simulink model "lidar_webcam_Bayes"  (Simulink 7.3)
settings: Solver=FixedStepDiscrete  StartTime=0.0  StopTime=inf  MaxStep=0.2  RelTol=1e-3
libraries: dspmtrx3 x2, simulink x1, vipstatistics x1, dspstat3 x1
(part 1 of 2)
settings Model: Creator=gclayton  LastModifiedBy=wildcat
settings DebuggingCC: InheritedTsInSrcMsg=none
settings RTWCC: SystemTargetFile=rlnx.tlc  GenCodeOnly=on  TemplateMakefile=rlnx_ubuntu.tmf  Description=Linux Real-Time Target  ProcessScript=rlnx_make_rtw_hook
settings RTWCC: CustomInclude=|
  | /usr/local/include/opencv/
  | /usr/local/include/
settings CodeAppCC: GenerateComments=off  SimulinkBlockComments=off
settings STFCustomTargetCC: ModelReferenceCompliant=off  MatFileLogging=on  SystemTargetFile=rlnx.tlc
settings GRTTargetCC: ModelReferenceCompliant=off  ParMdlRefBuildCompliant=off  CompOptLevelCompliant=off
settings CustomProperty: DataType=string  Value=-lm -ldl /usr/local/lib/libopencv_highgui.so.2.4 /usr/local/lib/libopencv_core.so.2.4 /usr/local/lib/libopencv_imgproc.so.2.4 -lc_urg -lc_urg_connection -lc_urg_system -lphidget21
settings EnumStrPairs: String=PC

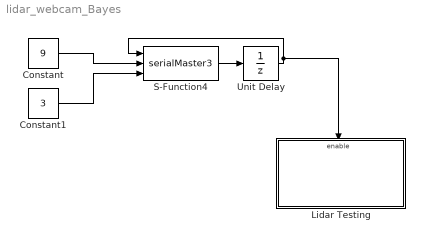
== system lidar_webcam_Bayes ==
  Constant : Constant  Value=9  OutDataTypeMode=int32  OutDataType=fixdt(1, 16)  OutScaling=2^0  OutDataTypeStr=int32
  Constant1 : Constant  Value=3  OutDataTypeMode=int32  OutDataType=fixdt(1, 16)  OutScaling=2^0  OutDataTypeStr=int32
  Lidar Testing : Subsystem  TreatAsAtomicUnit=on
  S-Function4 : S-Function  FunctionName=serialMaster3  EnableBusSupport=off
  Unit Delay : UnitDelay  SampleTime=-1
  wires:
  Constant1/1 -> S-Function4/3
  Constant/1 -> S-Function4/2
  S-Function4/1 -> Unit Delay/1
  Unit Delay/1 -> S-Function4/1, Lidar Testing/Enable

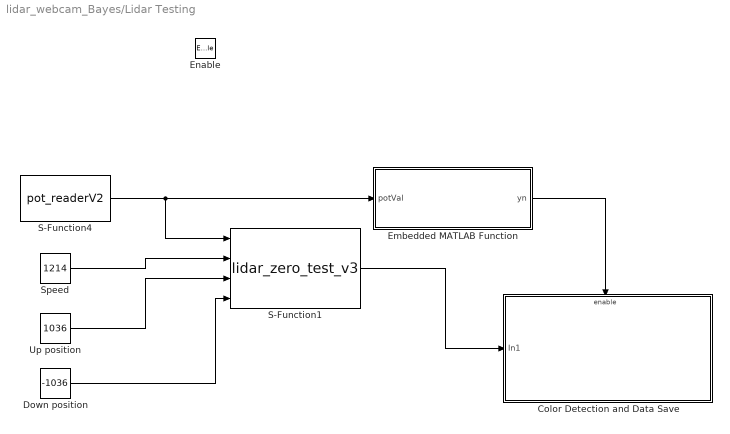
== system lidar_webcam_Bayes/Lidar Testing ==
  Enable : EnablePort
  Color Detection and Data Save : Subsystem  TreatAsAtomicUnit=on
  Down position : Constant  Value=-1036  OutDataType=fixdt(1, 16)  OutScaling=2^0
  Embedded MATLAB Function : Stateflow chart
  S-Function1 : S-Function  FunctionName=lidar_zero_test_v3  EnableBusSupport=off
  S-Function4 : S-Function  FunctionName=pot_readerV2  EnableBusSupport=off
  Speed : Constant  Value=1214  OutDataType=fixdt(1, 16)  OutScaling=2^0
  Up position : Constant  Value=1036  OutDataType=fixdt(1, 16)  OutScaling=2^0
  wires:
  Speed/1 -> S-Function1/2
  Up position/1 -> S-Function1/3
  Down position/1 -> S-Function1/4
  S-Function4/1 -> S-Function1/1, Embedded MATLAB Function/1(potVal)
  S-Function1/1 -> Color Detection and Data Save/1(In1)
  Embedded MATLAB Function/1(yn) -> Color Detection and Data Save/Enable

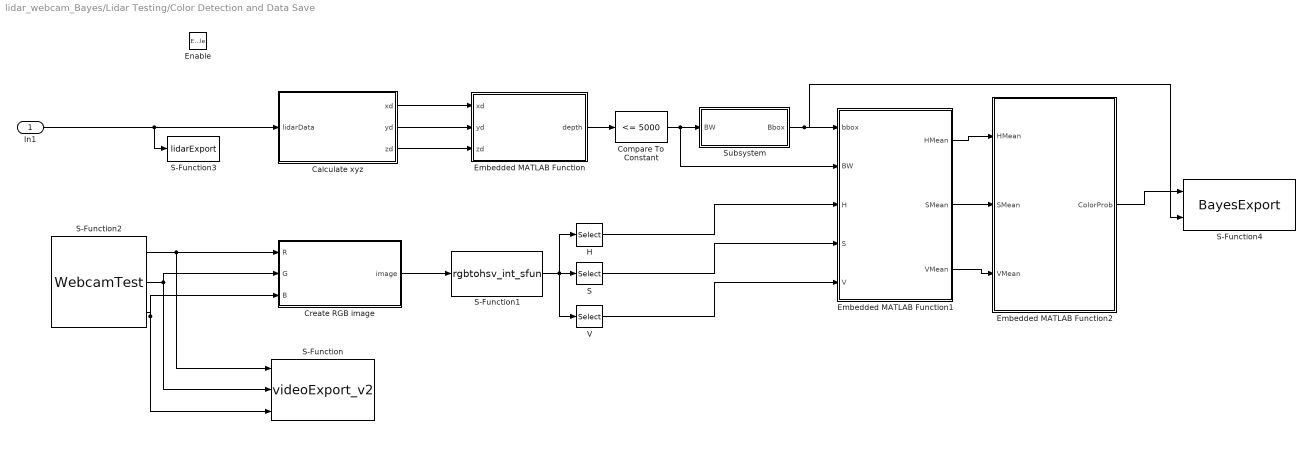
== system lidar_webcam_Bayes/Lidar Testing/Color Detection and Data Save ==
  In1 : Inport  OutDataType=fixdt(1, 16)  OutScaling=2^0
  Enable : EnablePort
  Calculate xyz : Stateflow chart
  Compare To Constant : simulink/Logic and Bit Operations/Compare To Constant  SystemSampleTime=-1  relop=<=  const=5000  LogicOutDataTypeMode=uint8  ZeroCross=off
  Create RGB image : Stateflow chart
  Embedded MATLAB Function : Stateflow chart
  Embedded MATLAB Function1 : Stateflow chart
  Embedded MATLAB Function2 : Stateflow chart
  H : Selector  NumberOfDimensions=3  InputPortWidth=3  IndexOptions=Select all,Select all,Index vector (dialog)  Indices=[1 3],1,1  OutputSizes=1,1,1
  S : Selector  NumberOfDimensions=3  InputPortWidth=3  IndexOptions=Select all,Select all,Index vector (dialog)  Indices=[1 3],1,2  OutputSizes=1,1,1
  S-Function : S-Function  FunctionName=videoExport_v2  EnableBusSupport=off
  S-Function1 : S-Function  FunctionName=rgbtohsv_int_sfun  EnableBusSupport=off
  S-Function2 : S-Function  FunctionName=WebcamTest  EnableBusSupport=off
  S-Function3 : S-Function  FunctionName=lidarExport  EnableBusSupport=off
  S-Function4 : S-Function  FunctionName=BayesExport  EnableBusSupport=off
  Subsystem : Subsystem
  V : Selector  NumberOfDimensions=3  InputPortWidth=3  IndexOptions=Select all,Select all,Index vector (dialog)  Indices=[1 3],1,3  OutputSizes=1,1,1
  wires:
  S-Function2/3 -> S-Function/3, Create RGB image/3(B)
  S-Function2/2 -> S-Function/2, Create RGB image/2(G)
  S-Function2/1 -> S-Function/1, Create RGB image/1(R)
  In1/1 -> S-Function3/1, Calculate xyz/1(lidarData)
  Create RGB image/1(image) -> S-Function1/1
  S-Function1/1 -> S/1, V/1, H/1
  Calculate xyz/1(xd) -> Embedded MATLAB Function/1(xd)
  Calculate xyz/2(yd) -> Embedded MATLAB Function/2(yd)
  Calculate xyz/3(zd) -> Embedded MATLAB Function/3(zd)
  Embedded MATLAB Function/1(depth) -> Compare To Constant/1
  Compare To Constant/1 -> Subsystem/1(BW), Embedded MATLAB Function1/2(BW)
  Subsystem/1(Bbox) -> Embedded MATLAB Function1/1(bbox), S-Function4/2
  H/1 -> Embedded MATLAB Function1/3(H)
  S/1 -> Embedded MATLAB Function1/4(S)
  V/1 -> Embedded MATLAB Function1/5(V)
  Embedded MATLAB Function1/3(VMean) -> Embedded MATLAB Function2/3(VMean)
  Embedded MATLAB Function1/2(SMean) -> Embedded MATLAB Function2/2(SMean)
  Embedded MATLAB Function1/1(HMean) -> Embedded MATLAB Function2/1(HMean)
  Embedded MATLAB Function2/1(ColorProb) -> S-Function4/1

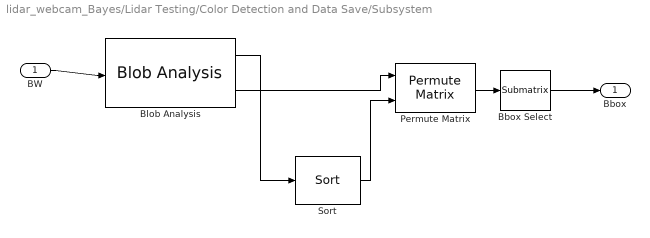
== system lidar_webcam_Bayes/Lidar Testing/Color Detection and Data Save/Subsystem ==
  BW : Inport  OutDataType=fixdt(1, 16)  OutScaling=2^0
  Bbox Select : dspmtrx3/Submatrix  RowSpan=One row  RowStartMode=First  RowStartIndex=1  RowEndMode=Last  RowEndIndex=1  ColSpan=All columns  ColStartMode=First  ColStartIndex=1  ColEndMode=Last  ColEndIndex=1
  Blob Analysis : vipstatistics/Blob Analysis  DialogController=vipDDGCreate  DialogControllerArgs=DataTag0  area=on  centroid=off  bBox=on  majorAxis=off  minorAxis=off  angle=off  eccentricity=off  equivDiameterSq=off  extent=off  perimeter=off  maxBlobs=20  warnIfNumBlobsExceeded=on  isCount=off  useMinArea=on  minArea=20  useMaxArea=off  maxArea=intmax('uint32')  excludeBorderBlob=off  outDT=double  isOutVarDim=off  isFill=on  fillValues=-1  conn=8  isLabel=off  outputMode=Binary point scaling  outputWordLength=32  outputFracLength=16  firstCoeffMode=Binary point scaling  firstCoeffWordLength=16  firstCoeffFracLength=14  secondCoeffMode=Binary point scaling  secondCoeffWordLength=32  secondCoeffFracLength=16  accumMode=Binary point scaling  accumWordLength=32  accumFracLength=0  prodOutputMode=Binary point scaling  prodOutputWordLength=32  prodOutputFracLength=16  roundingMode=Floor  overflowMode=off
  Permute Matrix : dspmtrx3/Permute Matrix  mode=Columns  ZeroOneIdxMode=One-based  errmode=Clip index  checkDims=off
  Sort : dspstat3/Sort  DialogController=dspDDGCreate  DialogControllerArgs=DataTag1  otype=Index  dir=Descending  sortAlg=Quick sort  roundingMode=Floor  overflowMode=off
  Bbox : Outport  OutDataType=fixdt(1, 16)  OutScaling=2^0
  wires:
  BW/1 -> Blob Analysis/1
  Blob Analysis/1 -> Sort/1
  Sort/1 -> Permute Matrix/2
  Blob Analysis/2 -> Permute Matrix/1
  Permute Matrix/1 -> Bbox Select/1
  Bbox Select/1 -> Bbox/1

== matlab function Lidar Testing/Embedded MATLAB Function ==
  data: potVal input double; yn output double
function yn = check_pot_val(potVal)
%#eml

% Pot value may initially be zero.
% Check for this and output a 1 or zero to 
% control whether the rest of model runs
if (potVal == 0)
    yn = 0;
else
    yn = 1;
end

== matlab function Lidar Testing/Color Detection and Data Save/Calculate xyz ==
  data: lidarData input double; xd output double; yd output double; zd output double
function [xd, yd, zd] = xyz_calc(lidarData)
%#eml

% Define variables based on gimbal system and scan pattern
ScanNum = 65;
DataLength = 1080*ScanNum;
h = 36.3;

% Define Data sizes
phim = zeros(1,DataLength);
thetam = zeros(1,DataLength);
distm = zeros(1,DataLength);
xd = zeros(1,DataLength);
yd = zeros(1,DataLength);
zd = zeros(1,DataLength);


%Define phi_rad: angles corresponding to one lidar scan
l = 1:1080;
phi_rad = (-45 + 0.25*l)*pi/180;

% Repeat thetam for number of scans
for i = 1:ScanNum
    % phi_start = 1+1080*(i-1);
    % phi_end = 1080*i;
    
    for j = 1 : 1080
        phi_val = 1080*(i-1) + j;
        phim(1,phi_val) = phi_rad(1,j);
    end
    % phim = [phim phi_rad]; 
end

% Theta changes from -45 to 45 degrees over the duration of the scan
theta_min = -45*pi/180;
theta_max = 45*pi/180;
theta_step = (theta_max - theta_min)/DataLength;
thetam = [theta_max : -theta_step : (theta_min+theta_step)];

% Distance matrix is directly from lidar data
distm = lidarData';

% Calculate x y and z
for k = 1:DataLength
    % Replace returned zeros with large number
    if (distm(1,k) == 0)
        distm = 30000;
    end
    xd(1,k) = distm(1,k)*cos(phim(1,k));
    yd(1,k) = distm(1,k)*sin(phim(1,k))*cos(thetam(1,k)) - h*sin(thetam(1,k));
    zd(1,k) = distm(1,k)*sin(phim(1,k))*sin(thetam(1,k)) + h*cos(thetam(1,k));
end

== matlab function Lidar Testing/Color Detection and Data Save/Create RGB image ==
  data: R input double; image output double; G input double; B input double
function image = create_image(R,G,B)
%#eml

% Create image from R G and B data
image = zeros(480,640,3);

image(:,:,1) = R;
image(:,:,2) = G;
image(:,:,3) = B;

== matlab function Lidar Testing/Color Detection and Data Save/Embedded MATLAB Function ==
  data: xd input double; depth output double; yd input double; zd input double
function depth   = scan2depth(xd, yd, zd )

%Written by Anderson Lebbad on June 19, 2014
%Last Edited:

%Converts xyz coordinates from the Lidar to the video frame. Outputs are
%uvd, where u is the position along the horizontal axis of the image, v is
%the position along the vertical axis of the image, and d is the depth of
%at that point - EXPECTS XYZ COORDINATES IN MILLIMETERS

%% Parse inputs
x = xd';
y = yd';
z = zd';

%% Transforms the xyz from lidar coordinate frame to image coordinate frame

% Translation vector (in meters)
t = [24;-113;38];

%Rotation angles
phi = (-90+6)*pi/180;
theta = 0*pi/180;

%Rotation about x-axis
Rx = [1 0 0; 0 cos(phi) sin(phi); 0 -sin(phi) cos(phi)];
%Rotation about y-axis
R = [cos(theta) 0 -sin(theta); 0 1 0; sin(theta) 0 cos(theta)]*Rx;

%Transformation matrix
T = [R t];

%-- Transformation:
Xc = T(1,1)*x+T(1,2)*y+T(1,3)*z+T(1,4);
Yc = T(2,1)*x+T(2,2)*y+T(2,3)*z+T(2,4);
Zc = T(3,1)*x+T(3,2)*y+T(3,3)*z+T(3,4);

%% Normalized Coordinates
Xn = Xc./Zc;
Yn = Yc./Zc;
Dp = sqrt(Xc.^2+Yc.^2+Zc.^2);

%% Distorted Coordinates

% Radial Distortions
RadDist = [0.069102182282360,-0.154608606024690,0.020241053576861];

% Tangential Distortions
TanDist = [-0.003474414312935,-0.001451647225947];

%-- Radial Vectors
r2 = Xn.^2+Yn.^2;
r6 = r2.^3;

%-- Transformation (second radial distortion term removed)
XradDist = Xn.*(1+RadDist(1).*r2+RadDist(3).*r6);
YradDist = Yn.*(1+RadDist(1).*r2+RadDist(3).*r6);
Xd = XradDist+2*TanDist(1).*Xn.*Yn+TanDist(2)*(r2+2*Xn.^2);
Yd = YradDist+TanDist(1).*(r2+2*Yn.^2)+2*TanDist(2).*Xn.*Yn;

%% Pixel Frame

% Intrinsic Matrix
K = [5.548581600685270e+02,0,0;0,5.523116000564020e+02,0;3.135858904821101e+02,2.190392333699872e+02,1];
KK = K';

%-- Transformation:
Xp = KK(1,1)*Xd+KK(1,2)*Yd+KK(1,3);
Yp = KK(2,1)*Xd+KK(2,2)*Yd+KK(2,3);

%% Interpolation to Pixel Coordinates

% image frame
u = 1:1:640;
v = 1:1:480;

% interpolation
[Ugrid, Vgrid] = meshgrid(u,v);
% image = griddata(Xp,Yp,Dp,Ugrid,Vgrid);
F = scatteredInterpolant(Xp,Yp,Dp);
image = F(Ugrid,Vgrid);
image = uint16(image);
depth = image;

end

== matlab function Lidar Testing/Color Detection and Data Save/Embedded MATLAB Function1 ==
  data: bbox input double; HMean output double; BW input double; H input double; S input double; V input double; SMean output double; VMean output double
function [HMean, SMean, VMean] = bbox_hist(bbox, BW, H, S, V)
%This function creates a histogram of the color region of a detected object
%identified in a binary image within a bounding box

%Initialize variables
pixels = 0;
HRunAve = 0;
SRunAve = 0;
VRunAve = 0;

%Parse bbox data
left = bbox(1);
right = left + bbox(3) - 1;
bottom = bbox(2);
top = bottom + bbox(4) - 1;

%Check to see if valid bbox is found
if left~=-1
    %Scan the detected region of the binary image and generate histograms
    for j=left:right
        for i=bottom:top
            if BW(i,j) == 1
                pixels = pixels + 1;
                HRunAve = ((pixels-1)/pixels)*HRunAve + (1/pixels)*double(H(i,j));
                SRunAve = ((pixels-1)/pixels)*SRunAve + (1/pixels)*double(S(i,j));
                VRunAve = ((pixels-1)/pixels)*VRunAve + (1/pixels)*double(V(i,j));
            end
        end
    end
end

%Means must be integers to use in Bayes Filter
HMean = uint8(HRunAve);
SMean = uint8(SRunAve);
VMean = uint8(VRunAve);

end
